simulink model "getResponeRobot_Odom_NEW"  (R2020a)
settings: Solver=FixedStepDiscrete  StartTime=0.0  StopTime=100  FixedStep=0.005  RelTol=1e-3
undefined symbols (not defined in the file or in its folder): CR, serial
libraries: mobileRoboticsLib x4, instrumentlib x2
settings Model: Creator=dangh  LastModifiedBy=dangh

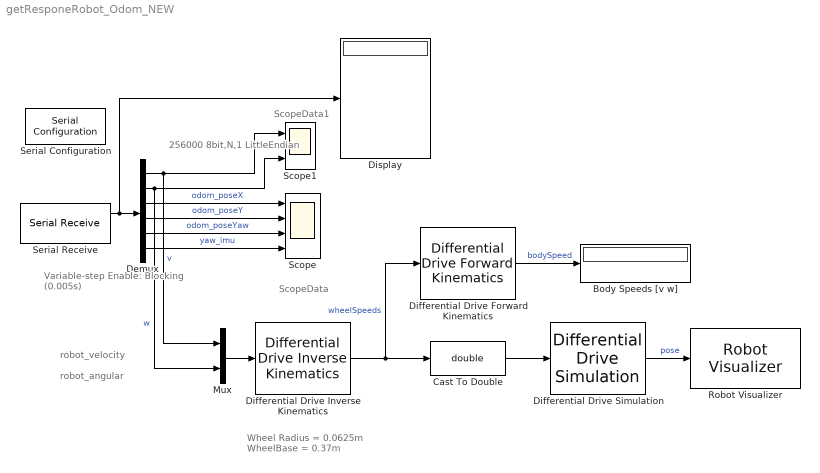
== system getResponeRobot_Odom_NEW ==
  note: Wheel Radius = 0.0625m
      | WheelBase = 0.37m
  note: robot_angular
  note: robot_velocity
  note: ScopeData1
  note: ScopeData
  note: 256000
      | 8bit,N,1
      | LittleEndian
  note: Variable-step
      | Enable: Blocking
      | (0.005s)
  Body Speeds [v w] : Display
  Cast To Double : DataTypeConversion  OutDataTypeStr=double
  Demux : Demux  Outputs=6
  Differential Drive Forward Kinematics : mobileRoboticsLib/Kinematic Models/Differential Drive/Differential Drive Forward Kinematics  wheelRadius=0.0625  wheelBase=0.37
      settings: SourceProductName=Mobile Robotics Simulation Library
  Differential Drive Inverse Kinematics : mobileRoboticsLib/Kinematic Models/Differential Drive/Differential Drive Inverse Kinematics  wheelRadius=0.0625  wheelBase=0.37
      settings: SourceProductName=Mobile Robotics Simulation Library
  Differential Drive Simulation : mobileRoboticsLib/Kinematic Models/Differential Drive/Differential Drive Simulation  wheelRadius=0.0625  wheelBase=0.37  initX=0  initY=0  initAngle=0  Ts=0.005
      settings: SourceProductName=Mobile Robotics Simulation Library
  Display : Display
  Mux : Mux  Inputs=2
  Robot Visualizer : mobileRoboticsLib/Environments/Robot Visualizer  Priority=99  robotRadius=0  showTrajectory=on  hasWaypoints=off  hasLidar=off  sensorOffset=[ 0 0 ]  scanAngles=scanAngles  hasObjDetector=off  objDetectorOffset=[ 0, 0 ]  objDetectorAngle=0  objDetectorFOV=pi/4  objDetectorMaxRange=5  objectColors=[ 1, 0, 0; 0, 1, 0; 0, 0, 1 ]  objectMarkers=s
      settings: SourceProductName=Mobile Robotics Simulation Library
  Scope : Scope  NumInputPorts=4
  Scope1 : Scope  NumInputPorts=2
  Serial Configuration : instrumentlib/Serial Configuration  Priority=-200000  ComPortMenu=COM8  ComPort=COM8  ObjConstructor=serial('COM8');  BaudRate=256000  DataBits=8  Parity=none  StopBits=1  FlowControl=none  Timeout=10  ByteOrder=LittleEndian
  Serial Receive : instrumentlib/Serial Receive  ComPortMenu=COM8  ComPort=COM8  ObjConstructor=serial('COM8');  Terminator=CR ('\r')  DataSize=6  DataType=single  EnableBlockingMode=off  ActionDataUnavailable=Output last received value  CustomValue=0  SampleTime=0.005
  wires:
  Serial Receive/1 -> Display/1, Demux/1
  Demux/1 -> Mux/1, Scope1/1  "v"
  Demux/2 -> Mux/2, Scope1/2  "w"
  Demux/3 -> Scope/1  "odom_poseX"
  Demux/4 -> Scope/2  "odom_poseY"
  Demux/5 -> Scope/3  "odom_poseYaw"
  Demux/6 -> Scope/4  "yaw_imu"
  Mux/1 -> Differential Drive Inverse Kinematics/1
  Differential Drive Inverse Kinematics/1 -> Differential Drive Forward Kinematics/1, Cast To Double/1  "wheelSpeeds"
  Differential Drive Forward Kinematics/1 -> Body Speeds [v w]/1  "bodySpeed"
  Cast To Double/1 -> Differential Drive Simulation/1
  Differential Drive Simulation/1 -> Robot Visualizer/1  "pose"
